simulink model "mod2_butterfly_scramble2"  (Simulink 8.1)
settings: Solver=FixedStepDiscrete  StartTime=0.0  StopTime=swpctrl.trantime  RelTol=1e-3
undefined symbols (not defined in the file or in its folder): DACctrl, Fs, modctrl, sinamp, sinfreq
libraries: dspsigops x6, simulink x4, dspsrcs4 x2
settings Model: Creator=amyles  LastModifiedBy=amyles
settings DataIOCC: LimitDataPoints=off  MaxDataPoints=50000
settings DebuggingCC: StrictBusMsg=Warning
settings SFSimCC: SimParseCustomCode=off

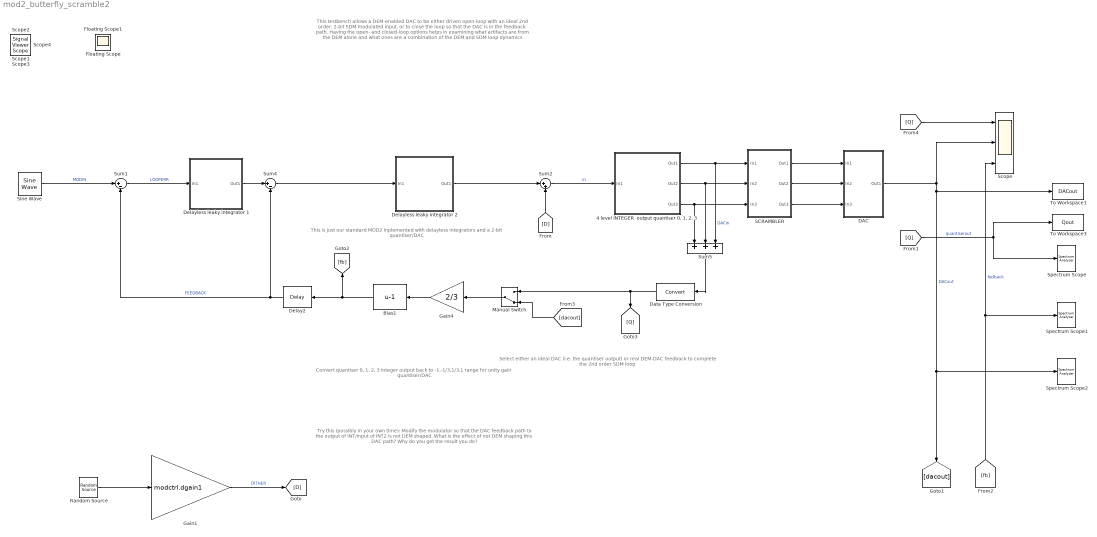
== system mod2_butterfly_scramble2 ==
  note: Convert quantiser 0, 1, 2, 3 integer
      | output back  to -1,-1/3,1/3,1 range for
      | unity gain quantiser/DAC
  note: Select either an ideal DAC
      | (i.e. the quantiser output) or real
      | DEM-DAC feedback to complete
      | the 2nd order SDM loop
  note: This testbench allows a DEM-enabled DAC to be either driven open-loop with an ideal 2nd order, 2-bit SDM modulated input,
      | or to close the loop so that the DAC is in the feedback path. Having the open- and closed-loop options helps in
      | examining what artifacts are from the DEM alone and what ones are a combination of the DEM and SDM loop dynamics
  note: This is just our standard MOD2 inplemented with delayless integrators and a 2-bit quantiser/DAC
  note: Try this (possibly in your own time):
      | Modify the modulator so that the DAC feedback path to the output of INT/input of INT2 is not DEM shaped.
      | What is the effect of not DEM shaping this DAC path? Why do you get the result you do?
  "4 level INTEGER  output quantiser 0, 1, 2, 3" : Subsystem
  Bias1 : Bias  Bias=-1
  DAC : Subsystem
  Data Type Conversion : DataTypeConversion
  Delay2 : dspsigops/Delay  InputProcessing=Columns as channels (frame based)  dly_unit=Samples  delay=1  ic_detail=off  dif_ic_for_ch=off  dif_ic_for_dly=off  ic=0  reset_popup=None
  Delayless leaky integrator 1 : Subsystem
  Delayless leaky integrator 2 : Subsystem
  Gain1 : Gain  Gain=modctrl.dgain1
      settings: AttributesFormatString=Dither level adjust
  Gain4 : Gain  Gain=2/3
      settings: AttributesFormatString=Integrator leakage
  Manual Switch : ManualSwitch  CurrentSetting=0
  Random Source : dspsrcs4/Random Source  SrcType=Uniform  NormMethod=Ziggurat  CltLength=12  MinVal=-1  MaxVal=1  MeanVal=0  VarVal=1  RepMode=Not repeatable  rawSeed=1  IsInherit=off  SampMode=Discrete  SampTime=1/Fs  SampFrame=1  DataType=Double  OutComplex=Real
      settings: AttributesFormatString=Dither source
  SCRAMBLER : Subsystem
  Scope : Scope  NumInputPorts=3
      settings: YMin=-5~-5~-5  YMax=5~5~5
  Sine Wave : dspsrcs4/Sine Wave  Amplitude=sinamp  Frequency=sinfreq  Phase=0  SampleMode=Discrete  OutComplex=Real  CompMethod=Trigonometric fcn  TableSize=Speed  SampleTime=1/Fs  SamplesPerFrame=1  ResetState=Restart at time zero  dataType=double  wordLen=16  udDataType=sfix(16)  fracBitsMode=Best precision  numFracBits=15  OutDataTypeStr=double  LastOutDataTypeStr=double
  Spectrum Scope : SpectrumAnalyzer
      settings: CopyFcn=scopeextensions.ScopeBlock.callback(gcbh, 'onBlockCopy', gcbh);  DeleteFcn=scopeextensions.ScopeBlock.callback(gcbh, 'onBlockDelete');  PreSaveFcn=scopeextensions.ScopeBlock.callback(gcbh, 'onModelSave');  NameChangeFcn=scopeextensions.ScopeBlock.callback(gcbh, 'onBlockRename');  CloseFcn=scopeextensions.ScopeBlock.callback(gcbh, 'onBlockClose');  PreDeleteFcn=scopeextensions.ScopeBlock.callback(gcbh, 'onBlockPreDelete');
  Spectrum Scope1 : SpectrumAnalyzer
      settings: CopyFcn=scopeextensions.ScopeBlock.callback(gcbh, 'onBlockCopy', gcbh);  DeleteFcn=scopeextensions.ScopeBlock.callback(gcbh, 'onBlockDelete');  PreSaveFcn=scopeextensions.ScopeBlock.callback(gcbh, 'onModelSave');  NameChangeFcn=scopeextensions.ScopeBlock.callback(gcbh, 'onBlockRename');  CloseFcn=scopeextensions.ScopeBlock.callback(gcbh, 'onBlockClose');  PreDeleteFcn=scopeextensions.ScopeBlock.callback(gcbh, 'onBlockPreDelete');
  Spectrum Scope2 : SpectrumAnalyzer
      settings: CopyFcn=scopeextensions.ScopeBlock.callback(gcbh, 'onBlockCopy', gcbh);  DeleteFcn=scopeextensions.ScopeBlock.callback(gcbh, 'onBlockDelete');  PreSaveFcn=scopeextensions.ScopeBlock.callback(gcbh, 'onModelSave');  NameChangeFcn=scopeextensions.ScopeBlock.callback(gcbh, 'onBlockRename');  CloseFcn=scopeextensions.ScopeBlock.callback(gcbh, 'onBlockClose');  PreDeleteFcn=scopeextensions.ScopeBlock.callback(gcbh, 'onBlockPreDelete');
  Sum1 : Sum  Inputs=|+-
      settings: AttributesFormatString=Modulator input\nloop servo error (input - fbk)
  Sum2 : Sum  Inputs=|++
  Sum4 : Sum  Inputs=|+-
  Sum5 : Sum  Inputs=+++
  To Workspace1 : ToWorkspace  VariableName=DACout  SampleTime=-1
  To Workspace3 : ToWorkspace  VariableName=Qout  SampleTime=-1
  Floating Scope : Scope
      settings: Floating=on
  Floating Scope1 : Scope
      settings: Floating=on  SaveName=ScopeData2
  Scope1 : SignalViewerScope  IOType=viewer  RefreshTime=0.035000
      settings: YMin=-2e+09  YMax=0
  Scope2 : SignalViewerScope  IOType=viewer  NumInputPorts=3  ZoomMode=xonly  RefreshTime=0.035000
      settings: YMin=-5~-5~-5  YMax=5~5~5
  Scope3 : SignalViewerScope  IOType=viewer  RefreshTime=0.035000
      settings: SaveName=ScopeData2
  Scope4 : SignalViewerScope  IOType=viewer  NumInputPorts=3  RefreshTime=0.035000
      settings: YMin=-5~-5~-5  YMax=5~5~5  SaveName=ScopeData3
  wires:
  Sum1/1 -> Delayless leaky integrator 1/1(In1)  "LOOPERR"
  Delay2/1 -> Sum1/2, Sum4/2  "FEEDBACK"
  Sine Wave/1 -> Sum1/1  "MODIN"
  Sum4/1 -> Delayless leaky integrator 2/1(In1)
  Random Source/1 -> Gain1/1
  Gain1/1 -> [D]  "DITHER"
  [D] -> Sum2/2
  Manual Switch/1 -> Gain4/1
  Bias1/1 -> Delay2/1, [fb]
  Gain4/1 -> Bias1/1
  Sum2/1 -> "4 level INTEGER  output quantiser 0, 1, 2, 3"/1(In1)  "in"
  Delayless leaky integrator 1/1(Out1) -> Sum4/1
  Delayless leaky integrator 2/1(Out1) -> Sum2/1
  Data Type Conversion/1 -> Manual Switch/1, [Q]
  [fb] -> Scope/3, Spectrum Scope1/1  "fedback"
  [dacout] -> Manual Switch/2
  [Q] -> To Workspace3/1, Spectrum Scope/1  "quantiserout"
  "4 level INTEGER  output quantiser 0, 1, 2, 3"/3(Out3) -> Sum5/1, SCRAMBLER/3(In3)
  "4 level INTEGER  output quantiser 0, 1, 2, 3"/2(Out2) -> Sum5/2, SCRAMBLER/2(In2)
  Sum5/1 -> Data Type Conversion/1
  "4 level INTEGER  output quantiser 0, 1, 2, 3"/1(Out1) -> Sum5/3, SCRAMBLER/1(In1)  "DACin"
  [Q] -> Scope/1
  SCRAMBLER/1(Out1) -> DAC/1(In1)
  SCRAMBLER/2(Out2) -> DAC/2(In2)
  SCRAMBLER/3(Out3) -> DAC/3(In3)
  DAC/1(Out1) -> Scope/2, To Workspace1/1, [dacout], Spectrum Scope2/1  "DACout"

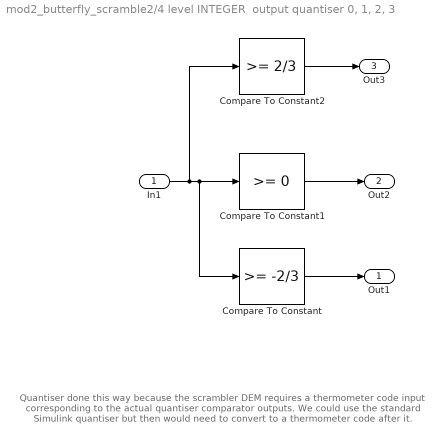
== system mod2_butterfly_scramble2/4 level INTEGER  output quantiser 0, 1, 2, 3 ==
  note: Quantiser done this way because the scrambler DEM
      | requires a thermometer code input corresponding to
      | the actual quantiser comparator outputs. We could use the
      | standard Simulink quantiser but then would need to convert
      | to a thermometer code after it.
  In1 : Inport
  Compare To Constant : simulink/Logic and Bit Operations/Compare To Constant  relop=>=  const=-2/3  OutDataTypeStr=uint8
  Compare To Constant1 : simulink/Logic and Bit Operations/Compare To Constant  relop=>=  const=0  OutDataTypeStr=uint8
  Compare To Constant2 : simulink/Logic and Bit Operations/Compare To Constant  relop=>=  const=2/3  OutDataTypeStr=uint8
  Out1 : Outport
  Out2 : Outport  Port=2
  Out3 : Outport  Port=3
  wires:
  In1/1 -> Compare To Constant/1, Compare To Constant1/1, Compare To Constant2/1
  Compare To Constant/1 -> Out1/1
  Compare To Constant1/1 -> Out2/1
  Compare To Constant2/1 -> Out3/1

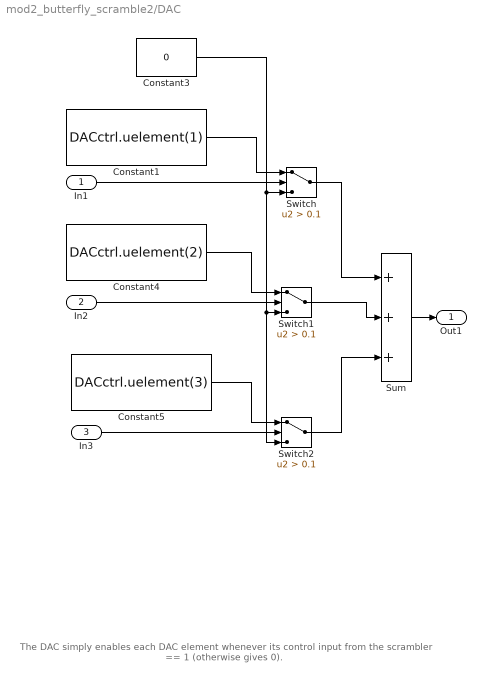
== system mod2_butterfly_scramble2/DAC ==
  note: The DAC simply enables each DAC element whenever its control
      | input from the scrambler == 1 (otherwise gives 0).
  In1 : Inport
  In2 : Inport  Port=2
  In3 : Inport  Port=3
  Constant1 : Constant  Value=DACctrl.uelement(1)  SampleTime=1/Fs
  Constant3 : Constant  Value=0  SampleTime=1/Fs
  Constant4 : Constant  Value=DACctrl.uelement(2)  SampleTime=1/Fs
  Constant5 : Constant  Value=DACctrl.uelement(3)  SampleTime=1/Fs
  Sum : Sum  Inputs=+++
  Switch : Switch  Criteria=u2 > Threshold  Threshold=0.1
  Switch1 : Switch  Criteria=u2 > Threshold  Threshold=0.1
  Switch2 : Switch  Criteria=u2 > Threshold  Threshold=0.1
  Out1 : Outport
  wires:
  Switch/1 -> Sum/1
  Switch1/1 -> Sum/2
  Switch2/1 -> Sum/3
  In1/1 -> Switch/2
  In2/1 -> Switch1/2
  Sum/1 -> Out1/1
  In3/1 -> Switch2/2
  Constant3/1 -> Switch/3, Switch1/3, Switch2/3
  Constant1/1 -> Switch/1
  Constant4/1 -> Switch1/1
  Constant5/1 -> Switch2/1

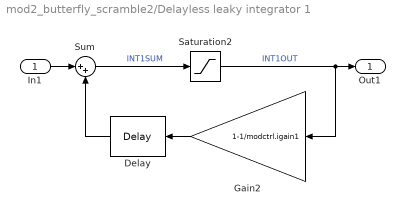
== system mod2_butterfly_scramble2/Delayless leaky integrator 1 ==
  In1 : Inport
  Delay : dspsigops/Delay  InputProcessing=Columns as channels (frame based)  dly_unit=Samples  delay=1  ic_detail=off  dif_ic_for_ch=off  dif_ic_for_dly=off  ic=0  reset_popup=None
  Gain2 : Gain  Gain=1-1/modctrl.igain1
      settings: AttributesFormatString=Integrator leakage
  Saturation2 : Saturate  UpperLimit=modctrl.isat1  LowerLimit=-(modctrl.isat1)
  Sum : Sum  Inputs=|++
      settings: AttributesFormatString=Integrator summer
  Out1 : Outport
  wires:
  Delay/1 -> Sum/2
  Sum/1 -> Saturation2/1  "INT1SUM"
  Gain2/1 -> Delay/1
  Saturation2/1 -> Gain2/1, Out1/1  "INT1OUT"
  In1/1 -> Sum/1

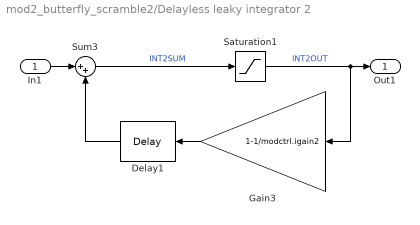
== system mod2_butterfly_scramble2/Delayless leaky integrator 2 ==
  In1 : Inport
  Delay1 : dspsigops/Delay  InputProcessing=Columns as channels (frame based)  dly_unit=Samples  delay=1  ic_detail=off  dif_ic_for_ch=off  dif_ic_for_dly=off  ic=0  reset_popup=None
  Gain3 : Gain  Gain=1-1/modctrl.igain2
      settings: AttributesFormatString=Integrator leakage
  Saturation1 : Saturate  UpperLimit=modctrl.isat2  LowerLimit=-(modctrl.isat2)
  Sum3 : Sum  Inputs=|++
      settings: AttributesFormatString=Integrator summer
  Out1 : Outport
  wires:
  Delay1/1 -> Sum3/2
  Sum3/1 -> Saturation1/1  "INT2SUM"
  Gain3/1 -> Delay1/1
  Saturation1/1 -> Gain3/1, Out1/1  "INT2OUT"
  In1/1 -> Sum3/1

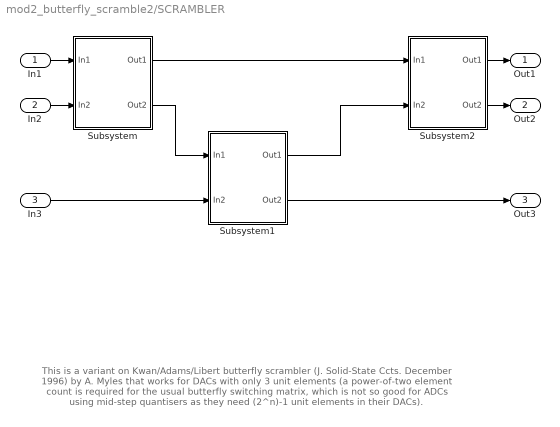
== system mod2_butterfly_scramble2/SCRAMBLER ==
  note: This is a variant on
      |
      | Kwan/Adams/Libert butterfly scrambler
      | (J. Solid-State Ccts. December 1996)
      |
      | by A. Myles that works for DACs with only 3 unit elements
      | (a power-of-two element count is required for the usual
      | butterfly switching matrix, which is not so good for
      | ADCs using mid-step quantisers as they need
      | (2^n)-1 unit elements in their DACs).
  In1 : Inport
  In2 : Inport  Port=2
  In3 : Inport  Port=3
  Subsystem : Subsystem
  Subsystem1 : Subsystem
      settings: AttributesFormatString=Non-standard\nswitching block
  Subsystem2 : Subsystem
  Out1 : Outport
  Out2 : Outport  Port=2
  Out3 : Outport  Port=3
  wires:
  Subsystem/1(Out1) -> Subsystem2/1(In1)
  In1/1 -> Subsystem/1(In1)
  Subsystem2/1(Out1) -> Out1/1
  In2/1 -> Subsystem/2(In2)
  Subsystem2/2(Out2) -> Out2/1
  In3/1 -> Subsystem1/2(In2)
  Subsystem1/2(Out2) -> Out3/1
  Subsystem/2(Out2) -> Subsystem1/1(In1)
  Subsystem1/1(Out1) -> Subsystem2/2(In2)

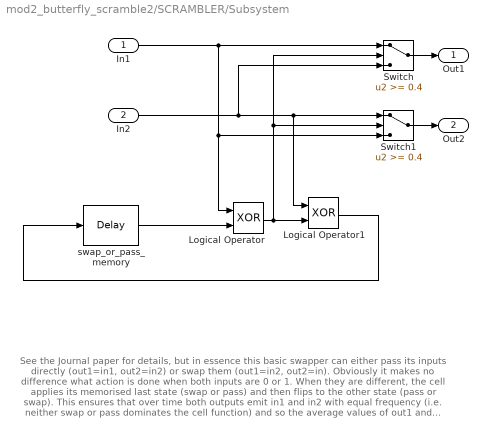
== system mod2_butterfly_scramble2/SCRAMBLER/Subsystem ==
  note: See the Journal paper for details, but in essence this basic swapper
      | can either pass its inputs directly (out1=in1, out2=in2) or swap
      | them (out1=in2, out2=in). Obviously it makes no difference what
      | action is done when both inputs are 0 or 1. When they are different,
      | the cell applies its memorised last state (swap or pass) and then flips
      | to the other state (pass or swap). This ensures that over time
      | both outputs emit in1 and in2 with equal frequency (i.e. neither
      | swap or pass dominates the cell function) and so the average values
      | of out1 and out2 are both (in1+in2)/2.
  In1 : Inport
  In2 : Inport  Port=2
  Logical Operator : Logic  Operator=XOR  AllPortsSameDT=off  OutDataTypeStr=boolean
  Logical Operator1 : Logic  Operator=XOR  AllPortsSameDT=off  OutDataTypeStr=boolean
  Switch : Switch  Threshold=0.4
  Switch1 : Switch  Threshold=0.4
  swap_or_pass_memory : dspsigops/Delay  InputProcessing=Inherited (this choice will be removed - see release notes)  dly_unit=Samples  delay=1  ic_detail=off  dif_ic_for_ch=off  dif_ic_for_dly=off  ic=0  reset_popup=None
  Out1 : Outport
  Out2 : Outport  Port=2
  wires:
  In1/1 -> Logical Operator/1, Switch1/3, Switch/1
  In2/1 -> Logical Operator1/1, Switch1/1, Switch/3
  Logical Operator/1 -> Switch/2, Switch1/2, Logical Operator1/2
  Logical Operator1/1 -> swap_or_pass_memory/1
  swap_or_pass_memory/1 -> Logical Operator/2
  Switch/1 -> Out1/1
  Switch1/1 -> Out2/1

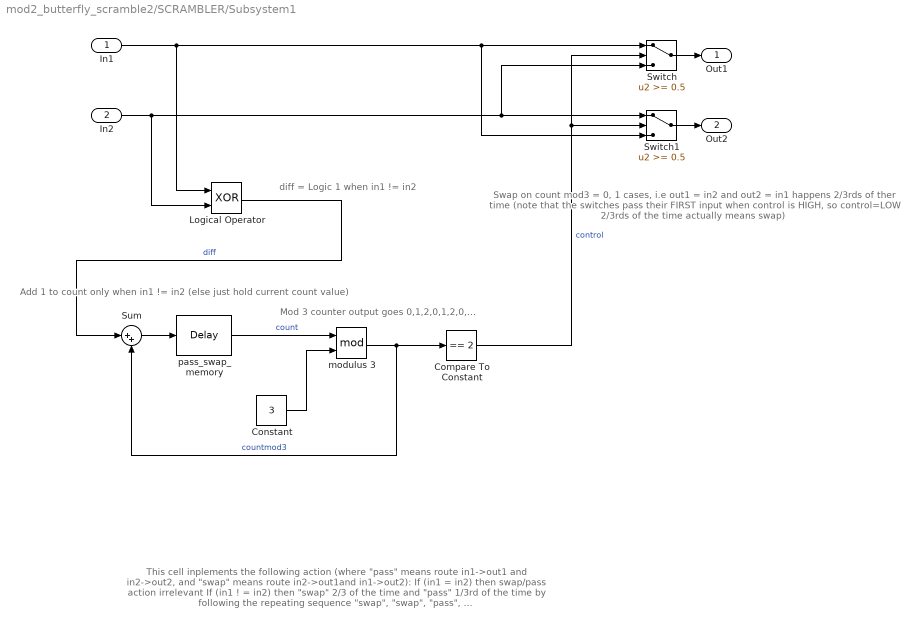
== system mod2_butterfly_scramble2/SCRAMBLER/Subsystem1 ==
  note: Add 1 to count only when in1 != in2
      | (else just hold current count value)
  note: This cell inplements the following action
      | (where "pass" means route in1->out1 and in2->out2,
      | and "swap" means route in2->out1and in1->out2):
      |
      | If (in1 = in2) then swap/pass action irrelevant
      |
      | If (in1 ! = in2) then "swap" 2/3 of the time and "pass"
      | 1/3rd of the time by following the repeating sequence
      | "swap", "swap", "pass", ...
  note: diff = Logic 1 when in1 != in2
  note: Mod 3 counter output goes 0,1,2,0,1,2,0,...
  note: Swap on count mod3 = 0, 1 cases,
      | i.e out1 = in2 and out2 = in1
      | happens 2/3rds of ther time
      | (note that the switches pass
      | their FIRST input when control
      | is HIGH, so control=LOW 2/3rds
      | of the time actually means swap)
  In1 : Inport
  In2 : Inport  Port=2
  Compare To Constant : simulink/Logic and Bit Operations/Compare To Constant  relop===  const=2  OutDataTypeStr=boolean
  Constant : Constant  Value=3
  Logical Operator : Logic  Operator=XOR  AllPortsSameDT=off  OutDataTypeStr=boolean
  Sum : Sum  Inputs=|++
  Switch : Switch  Threshold=0.5
  Switch1 : Switch  Threshold=0.5
  modulus 3 : Math  Operator=mod  SaturateOnIntegerOverflow=on
  pass_swap_memory : dspsigops/Delay  InputProcessing=Inherited (this choice will be removed - see release notes)  dly_unit=Samples  delay=1  ic_detail=off  dif_ic_for_ch=off  dif_ic_for_dly=off  ic=0  reset_popup=None
  Out1 : Outport
  Out2 : Outport  Port=2
  wires:
  Switch1/1 -> Out2/1
  Switch/1 -> Out1/1
  In2/1 -> Switch/3, Switch1/1, Logical Operator/2
  In1/1 -> Switch/1, Switch1/3, Logical Operator/1
  Logical Operator/1 -> Sum/1  "diff"
  Constant/1 -> modulus 3/2
  modulus 3/1 -> Compare To Constant/1, Sum/2  "countmod3"
  pass_swap_memory/1 -> modulus 3/1  "count"
  Sum/1 -> pass_swap_memory/1
  Compare To Constant/1 -> Switch1/2, Switch/2  "control"

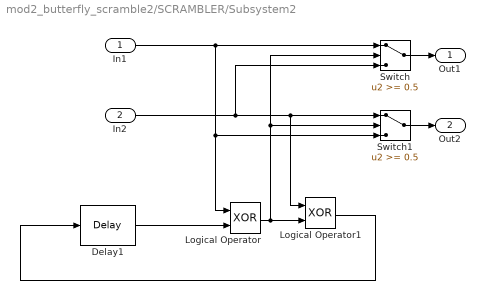
== system mod2_butterfly_scramble2/SCRAMBLER/Subsystem2 ==
  In1 : Inport
  In2 : Inport  Port=2
  Delay1 : dspsigops/Delay  InputProcessing=Inherited (this choice will be removed - see release notes)  dly_unit=Samples  delay=1  ic_detail=off  dif_ic_for_ch=off  dif_ic_for_dly=off  ic=0  reset_popup=None
  Logical Operator : Logic  Operator=XOR  AllPortsSameDT=off  OutDataTypeStr=boolean
  Logical Operator1 : Logic  Operator=XOR  AllPortsSameDT=off  OutDataTypeStr=boolean
  Switch : Switch  Threshold=0.5
  Switch1 : Switch  Threshold=0.5
  Out1 : Outport
  Out2 : Outport  Port=2
  wires:
  Switch1/1 -> Out2/1
  Switch/1 -> Out1/1
  Delay1/1 -> Logical Operator/2
  Logical Operator1/1 -> Delay1/1
  Logical Operator/1 -> Logical Operator1/2, Switch1/2, Switch/2
  In2/1 -> Switch/3, Switch1/1, Logical Operator1/1
  In1/1 -> Switch/1, Switch1/3, Logical Operator/1
